simulink model "PMSM_modular_vector_control_sim"  (R2019a)
settings: Solver=ode4  StartTime=0.0  StopTime=Tfinal  FixedStep=Ts  RelTol=1e-3  EnableMultiTasking=on
values from neighbouring files (symbols this model uses):
  Cdc = 150e-6    (= 0.00015)    [PMSM_modular_vector_control_sim_parameters.m]    (also in PMSM_vector_control_single_parameters.m)
  IdPIDmax = Vdcm/5    (= 20)    [PMSM_modular_vector_control_sim_parameters.m]    (also in PMSM_vector_control_single_parameters.m = 54)
  IdPIDmin = -Vdcm/5    (= -20)    [PMSM_modular_vector_control_sim_parameters.m]    (also in PMSM_vector_control_single_parameters.m = -54)
  IdrefM1 = 0    [PMSM_modular_vector_control_sim_parameters.m]
  IdrefM2 = 0    [PMSM_modular_vector_control_sim_parameters.m]
  Inertia = 1e-2    (= 0.01)    [PMSM_modular_vector_control_sim_parameters.m]    (also in PMSM_vector_control_single_parameters.m)
  IqPIDmax = Vdcm-10    (= 90)    [PMSM_modular_vector_control_sim_parameters.m]    (also in PMSM_vector_control_single_parameters.m = 260)
  IqPIDmin = -(Vdcm-10)    (= -90)    [PMSM_modular_vector_control_sim_parameters.m]    (also in PMSM_vector_control_single_parameters.m = -260)
  IrefOverTref = MotorSpeedRad/(EfRated*3)    (= 0.261799387799)    [PMSM_modular_vector_control_sim_parameters.m]    (also in PMSM_vector_control_single_parameters.m)
  LoadTorque1 = 2    [PMSM_modular_vector_control_sim_parameters.m]    (also in PMSM_vector_control_single_parameters.m = 30)
  LoadTorque2 = 2    [PMSM_modular_vector_control_sim_parameters.m]    (also in PMSM_vector_control_single_parameters.m = 20)
  LoadTorqueStepTime = 3    [PMSM_modular_vector_control_sim_parameters.m]    (also in PMSM_vector_control_single_parameters.m = 0.5)
  MechanicalLoadTorque1 = 2    [PMSM_modular_vector_control_sim_parameters.m]
  phase = [0 0 0 0]    [PMSM_modular_vector_control_sim_parameters.m]    (also in PMSM_vector_control_single_parameters.m)
  PMSMLoadResistance = 1e3    (= 1000)    [PMSM_modular_vector_control_sim_parameters.m]
  PolePairs = 10    [PMSM_modular_vector_control_sim_parameters.m]    (also in PMSM_vector_control_single_parameters.m)
  Rin = 1e-3    (= 0.001)    [PMSM_modular_vector_control_sim_parameters.m]    (also in PMSM_vector_control_single_parameters.m)
  Ripth = 0.1    [PMSM_modular_vector_control_sim_parameters.m]    (also in PMSM_vector_control_single_parameters.m)
  Rs = 321e-3    (= 0.321)    [PMSM_modular_vector_control_sim_parameters.m]    (also in PMSM_vector_control_single_parameters.m)
  SpeedPIDmax = 20    [PMSM_modular_vector_control_sim_parameters.m]    (also in PMSM_vector_control_single_parameters.m = 60)
  SpeedPIDmin = -20    [PMSM_modular_vector_control_sim_parameters.m]    (also in PMSM_vector_control_single_parameters.m = -60)
  SpeedRef1 = 200    [PMSM_modular_vector_control_sim_parameters.m]    (also in PMSM_vector_control_single_parameters.m = 600)
  SpeedRef2 = 100    [PMSM_modular_vector_control_sim_parameters.m]    (also in PMSM_vector_control_single_parameters.m = 200)
  SpeedRefStepTime = 6    [PMSM_modular_vector_control_sim_parameters.m]    (also in PMSM_vector_control_single_parameters.m = 0.5)
  Ts = 1000e-9    (= 1e-06)    [PMSM_modular_vector_control_sim_parameters.m]    (also in PMSM_vector_control_single_parameters.m)
  Vdc = 200    [PMSM_modular_vector_control_sim_parameters.m]    (also in PMSM_vector_control_single_parameters.m = 270)
  Vin = Vdc + Rin*(Pout/Vdc)    (= 200.01)    [PMSM_modular_vector_control_sim_parameters.m]    (also in PMSM_vector_control_single_parameters.m = 270.007407407)
  ViscousFriction = 1e-3    (= 0.001)    [PMSM_modular_vector_control_sim_parameters.m]    (also in PMSM_vector_control_single_parameters.m)
undefined symbols (not defined in the file or in its folder): Lload, Rload
libraries: powerlib x41, powerlib_meascontrol x33, fl_lib x12, simulink x9, nesl_utility x8, sdl_lib x2
(part 2 of 2)

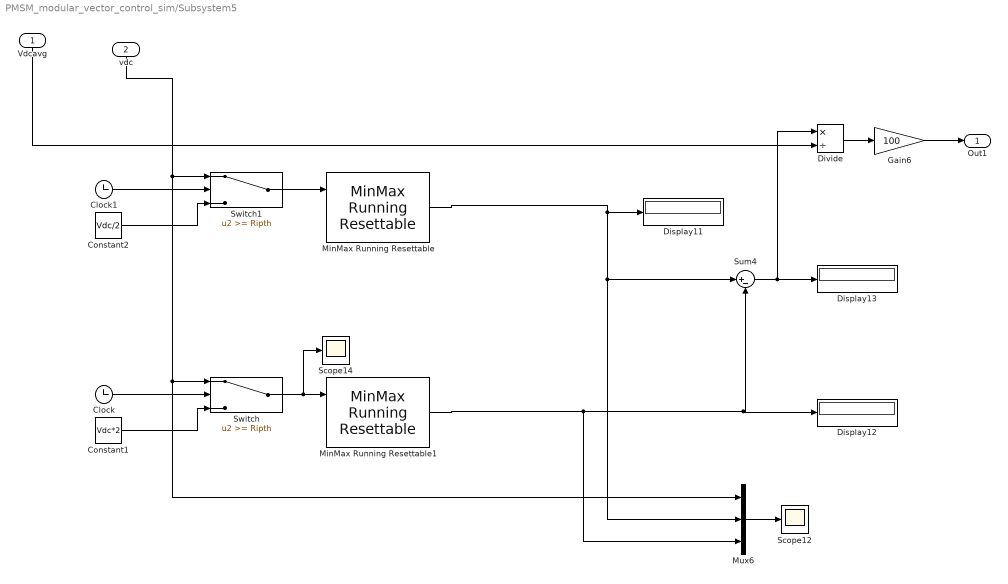
== system PMSM_modular_vector_control_sim/Subsystem5 ==
  Vdcavg : Inport
  vdc : Inport  Port=2
  Clock : Clock
  Clock1 : Clock
  Constant1 : Constant  Value=Vdc*2  SampleTime=Ts
  Constant2 : Constant  Value=Vdc/2  SampleTime=Ts
  Display11 : Display
  Display12 : Display
  Display13 : Display
  Divide : Product  Inputs=*/
  Gain6 : Gain  Gain=100
  MinMax Running Resettable : simulink/Math Operations/MinMax Running Resettable  Function=max  vinit=0.0
  MinMax Running Resettable1 : simulink/Math Operations/MinMax Running Resettable  Function=min  vinit=Vdc*4
  Mux6 : Mux  Inputs=3
  Scope12 : Scope
  Scope14 : Scope
  Sum4 : Sum  Inputs=|+-
  Switch : Switch  Threshold=Ripth
  Switch1 : Switch  Threshold=Ripth
  Out1 : Outport
  wires:
  MinMax Running Resettable/1 -> Display11/1, Mux6/2, Sum4/1
  Clock/1 -> Switch/2
  Gain6/1 -> Out1/1
  Constant1/1 -> Switch/3
  MinMax Running Resettable1/1 -> Mux6/3, Display12/1, Sum4/2
  Switch/1 -> Scope14/1, MinMax Running Resettable1/1
  Sum4/1 -> Divide/1, Display13/1
  Divide/1 -> Gain6/1
  Mux6/1 -> Scope12/1
  Vdcavg/1 -> Divide/2
  vdc/1 -> Switch1/1, Mux6/1, Switch/1
  Switch1/1 -> MinMax Running Resettable/1
  Clock1/1 -> Switch1/2
  Constant2/1 -> Switch1/3
